simulink model "vending_machine"  (R2019a)
settings: Solver=FixedStepAuto  StartTime=0.0  StopTime=inf  FixedStep=1  RelTol=1e-3
settings Model: Creator=anton  LastModifiedBy=anton

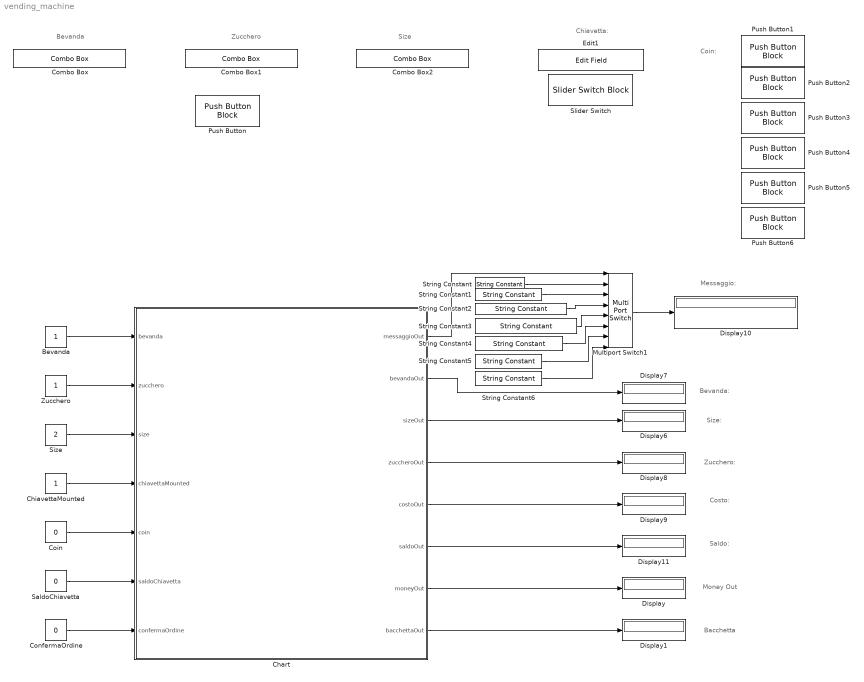
== system vending_machine ==
  note: Bacchetta
  note: Money Out
  note: Chiavetta:
  note: Coin:
  note: Messaggio:
  note: Saldo:
  note: Costo:
  note: Zucchero:
  note: Bevanda:
  note: Size:
  note: Size
  note: Zucchero
  note: Bevanda
  Bevanda : Constant
  Chart : Stateflow chart  BlockKeywords=__PRM__SERIALIZED__DATA__:Stateflow Chart,Stateflow Diagram  TreatAsAtomicUnit=on
  ChiavettaMounted : Constant
  Coin : Constant  Value=0
  Combo Box : ComboBox  LabelPosition=Hide  SelectedLabel=Caffe
      settings: Values={{'-', 'Caffe', 'The', 'Cioccolata'}, [0 1 2 3]}
  Combo Box1 : ComboBox  LabelPosition=Hide  SelectedLabel=Low
      settings: Values={{'-', 'Low', 'Medium', 'High'}, [0 1 2 3]}
  Combo Box2 : ComboBox  LabelPosition=Hide  SelectedLabel=Medium
      settings: Values={{'-', 'Small', 'Medium', 'Large'}, [0 1 2 3]}
  ConfermaOrdine : Constant  Value=0
  Display{,1,6..11} (8 alike) : Display
  Edit1 : EditField  LabelPosition=Hide  ShowInitialText=on  Alignment=Center
  Multiport Switch1 : MultiPortSwitch  Inputs=7
  Push Button : PushButtonBlock  ButtonText=Conferma
  Push Button1 : PushButtonBlock  ButtonText=0.05€  OnValue=0.05
  Push Button2 : PushButtonBlock  ButtonText=0.1€  OnValue=0.1
  Push Button3 : PushButtonBlock  ButtonText=0.2€  OnValue=0.2
  Push Button4 : PushButtonBlock  ButtonText=0.5€  OnValue=0.5
  Push Button5 : PushButtonBlock  ButtonText=1€
  Push Button6 : PushButtonBlock  ButtonText=2€  OnValue=2
  SaldoChiavetta : Constant  Value=0
  Size : Constant  Value=2
  Slider Switch : SliderSwitchBlock
      settings: Values={{'Off', 'On'}, [0 1]}
  String Constant : StringConstant  String="\"Benvenuto\""
  String Constant1 : StringConstant  String="\"Inserisci Denaro\""
  String Constant2 : StringConstant  String="\"Chiavetta Riconosciuta\""
  String Constant3 : StringConstant  String="\"Credito Insufficiente, perfavore ricarica\""
  String Constant4 : StringConstant  String="\"Moneta inserita non valida\""
  String Constant5 : StringConstant  String="\"Credito sufficiente, erogo prodotto\""
  String Constant6 : StringConstant  String="\"Ritirare il prodotto\""
  "Zucchero " : Constant
  wires:
  Bevanda/1 -> Chart/1(bevanda)
  "Zucchero "/1 -> Chart/2(zucchero)
  Size/1 -> Chart/3(size)
  ChiavettaMounted/1 -> Chart/4(chiavettaMounted)
  Coin/1 -> Chart/5(coin)
  SaldoChiavetta/1 -> Chart/6(saldoChiavetta)
  Chart/2(bevandaOut) -> Display7/1
  Chart/3(sizeOut) -> Display6/1
  Chart/4(zuccheroOut) -> Display8/1
  Chart/5(costoOut) -> Display9/1
  Chart/6(saldoOut) -> Display11/1
  Chart/1(messaggioOut) -> Multiport Switch1/1
  String Constant/1 -> Multiport Switch1/2
  Multiport Switch1/1 -> Display10/1
  String Constant1/1 -> Multiport Switch1/3
  ConfermaOrdine/1 -> Chart/7(confermaOrdine)
  String Constant2/1 -> Multiport Switch1/4
  String Constant3/1 -> Multiport Switch1/5
  Chart/7(moneyOut) -> Display/1
  String Constant4/1 -> Multiport Switch1/6
  String Constant5/1 -> Multiport Switch1/7
  String Constant6/1 -> Multiport Switch1/8
  Chart/8(bacchettaOut) -> Display1/1

== stateflow chart vending_machine/Chart ==
  state Idle
    entry:
    messaggioOut=1;
    bevandaOut=0;
    sizeOut=0;
    zuccheroOut=0;
    costoOut=0;
    bacchettaOut=0;
    saldoOut=0;
    moneyOut=0;
    during:
    messaggioOut=1;
    costoOut=0;
    saldoOut=0;
    pause(1);
  state OrderConfirmed
    messaggioOut=2;
    costoOut=COSTO_BEVANDA;
    pause(1);
  state Gadged
    messaggioOut=3;
    saldoOut=saldoChiavetta;
    pause(1);
  state CreditoInsufficiente
    messaggioOut=4;
    pause(1);
  state Detection
    actualCoin=coin;
    if actualCoin==0.05 || actualCoin==0.1 || actualCoin==0.2 || actualCoin ==0.5 || actualCoin==1 || actualCoin==2
    isConfirmed=true;
    if rand(1)>1
    isConfirmed = false
    end
    else
    isConfirmed=false;
    end
  state CoinAcceptedCash
    entry:
    saldoTmp=saldoOut+actualCoin;
    actualCoin=0;
    during:
    saldoOut=saldoTmp;
  state CoinAcceptedChiavetta
    entry:
    saldoTmp=saldoOut+actualCoin;
    actualCoin=0;
    during:
    saldoOut=saldoTmp;
  state CoinRefused
    messaggioOut=5;
    moneyOut=actualCoin;
    actualCoin=0;
    pause(1)
  state ErogaProdotto
    messaggioOut=7;
    bevandaOut=bevanda;
    sizeOut=size;
    zuccheroOut=zucchero;
    if zucchero==1
    bacchettaOut=0;
    else
    bacchettaOut=1;
    end
    pause(1);
  state CreditoSufficiente
    messaggioOut=6;
    if chiavettaMounted==1
    saldoOut = saldoOut-COSTO_BEVANDA;
    end
    if chiavettaMounted==0
    moneyOut=saldoOut-COSTO_BEVANDA;
    saldoOut=0;
    end
  (default) -> Idle
  ErogaProdotto -> Idle : [after(10,sec)]
  CreditoInsufficiente -> Idle [order 1] : [after(10,sec)]
  Detection -> Idle [order 2] : [after(10,sec)]
  Idle -> OrderConfirmed : [confermaOrdine==1 && bevanda~=0 && zucchero~=0 && size~=0]
  OrderConfirmed -> Idle [order 1] : [after(10,sec)]
  OrderConfirmed -> Detection [order 3] : [coin>0]
  OrderConfirmed -> Gadged [order 2] : [chiavettaMounted==1]
  Gadged -> CreditoSufficiente [order 1] : [saldoChiavetta>=COSTO_BEVANDA]
  CoinRefused -> Gadged [order 1] : [chiavettaMounted==1]
  Gadged -> CreditoInsufficiente [order 2] : [saldoChiavetta<COSTO_BEVANDA]
  CoinRefused -> CreditoInsufficiente [order 3] : [chiavettaMounted == 0]
  CreditoInsufficiente -> Detection [order 2] : [coin>0]
  CoinAcceptedCash -> Detection [order 1] : [coin>0]
  Detection -> CoinAcceptedCash [order 1] : [isConfirmed==true && chiavettaMounted==0]
  Detection -> CoinAcceptedChiavetta [order 3] : [isConfirmed==true && chiavettaMounted==1]
  CoinAcceptedChiavetta -> Detection [order 1] : [coin>0]
  Detection -> CoinRefused [order 4] : [isConfirmed==false]
  CoinRefused -> Detection [order 2] : [coin>0]
  CoinAcceptedChiavetta -> CreditoSufficiente [order 2] : [saldoOut>=COSTO_BEVANDA]
  CoinAcceptedCash -> CreditoSufficiente [order 2] : [saldoOut>=COSTO_BEVANDA]
  CreditoSufficiente -> ErogaProdotto
  data: bevanda input; zucchero input; size input; chiavettaMounted input; coin input; saldoChiavetta input; messaggioOut output; bevandaOut output; sizeOut output; zuccheroOut output; costoOut output; saldoOut output; confermaOrdine input; COSTO_BEVANDA local =0.5; moneyOut output; actualCoin local; isConfirmed local; saldoTmp local; bacchettaOut output
